simulink model "simulation"  (R2023a)
settings: Solver=VariableStepAuto  StartTime=0.0  StopTime=0.2  MaxStep=1e-5  RelTol=1e-3
settings Model: Creator=gabri  LastModifiedBy=gabri

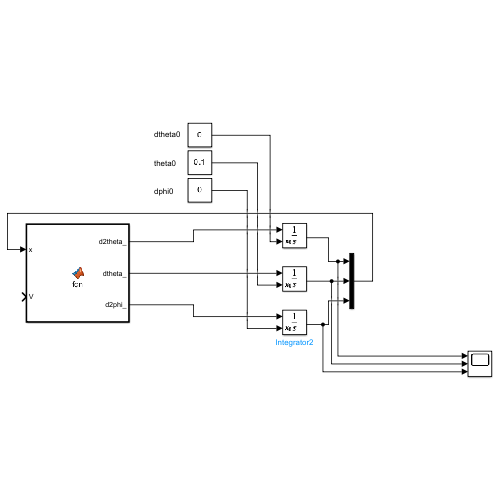
[thumbnail: Simulink's stored preview of the top-level diagram]
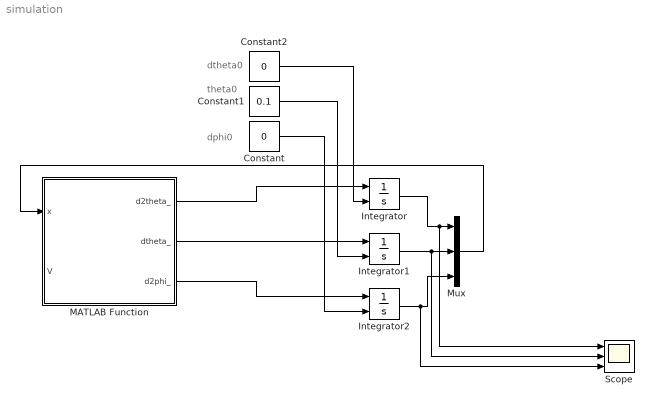
== system simulation ==
  note: dtheta0
  note: theta0
  note: dphi0
  Constant : Constant  Value=0
  Constant1 : Constant  Value=0.1
  Constant2 : Constant  Value=0
  Integrator : Integrator  InitialConditionSource=external
  Integrator1 : Integrator  InitialConditionSource=external
  Integrator2 : Integrator  InitialConditionSource=external
  MATLAB Function : MATLAB Function  TreatAsAtomicUnit=on
  Mux : Mux  Inputs=3
  Scope : Scope  NumInputPorts=3
  wires:
  Constant/1 -> Integrator2/2
  Constant1/1 -> Integrator1/2
  Constant2/1 -> Integrator/2
  MATLAB Function/1(d2theta_) -> Integrator/1
  MATLAB Function/2(dtheta_) -> Integrator1/1
  MATLAB Function/3(d2phi_) -> Integrator2/1
  Integrator/1 -> Scope/1, Mux/1
  Integrator2/1 -> Scope/3, Mux/3
  Mux/1 -> MATLAB Function/1(x)
  Integrator1/1 -> Scope/2, Mux/2

== matlab function simulation/MATLAB Function ==
  data: x input size=3; d2theta_ output size=1; V input size=1; dtheta_ output size=1; d2phi_ output size=1
function [d2theta_, dtheta_, d2phi_]  = fcn(x, V)
dtheta = x(1); 
theta = x(2);
dphi = x(3);

rw = 3.5e-2;
mb = 9.19e-1;
mw = 4.6e-2;
Ib = 4.068e-3;
Iw = 5.612e-5;
kv = 6.488e-3;
g = 9.801;
l = 6.247e-2;
kt = 6.538e-1; 
kw = 7.816e-1;
R = 6.05;

detA = 1/( (Ib+mb*l^2)*(mb*rw^2 + mw*rw^2 + Iw) - (mb*rw*l*cos(theta))^2);
iA11 = detA*(mb*rw^2 + mw*rw^2 + Iw);
iA12 = detA*(-mb*rw*l*cos(theta)); 
iA21 = iA12;
iA22 = detA*(Ib+mb*l^2);

iA1 = [iA11 iA21];
iA2 = [iA12 iA22];

k_V = zeros(2, 1);
k_dtheta_dphi = zeros(2, 1);
k_sin_theta = zeros(2, 1);
k_d2theta_sin = zeros(2, 1);

for i = 1:2
    k_V(i)              = (iA2(i)-iA1(i))*(2*kt/R);
    k_dtheta_dphi(i)    = (iA2(i)-iA1(i))*(2*kv + 2*kt*kw/R);
    k_sin_theta(i)      = iA1(i)*mb*g*l*sin(theta);
    k_d2theta_sin(i)    = iA2(i)*mb*rw*l*(dtheta^2)*sin(theta);
end


d2theta_ = k_V(1)*V + k_dtheta_dphi(1)*(dtheta-dphi) + k_sin_theta(1) + k_d2theta_sin(1);
dtheta_ = dtheta;
d2phi_ = k_V(2)*V + k_dtheta_dphi(2)*(dtheta-dphi) + k_sin_theta(2) + k_d2theta_sin(2);
